simulink model "GridFormingConverter"  (R2024b)
settings: Solver=ode1be  StartTime=0.0  StopTime=simulationTime  FixedStep=gridInverter.vsm.samplingTime  MaxStep=gridInverter.vsm.samplingTime  RelTol=1e-3  AbsTol=1e-3
PreLoadFcn:
  | % Parameterize the model
  | GridFormingConverterInputParameters;
  | GFLParameters;
PostLoadFcn:
  | GridFormingConverterTestCondition;
  | GFLParameters;
undefined symbols (not defined in the file or in its folder): base, ConvCtrl, ConvPlt, DiscIntNeverNeededParam, Discrete, Fault, gcbh, GFMGFLSelect, grid, gridInverter, HMI, localSolverSampleTime, magnitude, PlantSim, scrFactorRg, scrFactorXg, sps, sps_rtmsupport, spsPLL3phModel, transformer, TransmissionLine, Trf
libraries: powerlib_extras x39, ee_lib x21, eeGeneralControl x19, nesl_utility x16, simulink x13, eeTransforms x10, fl_lib x7, spsSecondOrderFilterLib x4, spsabctodq0Lib x4, spsPower3phInstantaneousLib x3, spsMeanLib x2, eeSinGeneratorThreePhase x1
(part 2 of 6)

== system GridFormingConverter/Transformer 415 V//11 kV ==
  Circuit Breaker : ee_lib/Switches & Breakers/Circuit Breaker (Three-Phase)  R_closed=0.001 Ohm  G_open=1e-6 1/Ohm  threshold=0.5 V  breaker_behavior=ee.enum.switches.breakerBehavior.zeroCrossingEnable
      settings: InternalSimscapePortConfiguration="{\"Bottom\":[],\"Left\":[{\"id\":\"vT\",\"label\":\"vT\",\"type\":\"input\"},{\"id\":\"N1\",\"label\":\"~1\",\"type\":\"foundation.electrical.three_phase\"}],\"Right\":[{\"id\":\"N2\",\"label\":\"~2\",\"type\":\"foundation.electrical.three_phase\"}],\"Top\":[]}"
  Circuit breaker : FromWorkspace  VariableName=testCondition.circuitBreakerTripSignalProfile  SampleTime=localSolverSampleTime  Interpolate=off  OutputAfterFinalValue=Holding final value
  Filter & Sensor : Subsystem
      mask Display: image('$imagefile'); % Use "Edit Image" on toolstrip to change.
  Simulink-PS Converter : nesl_utility/Simulink-PS Converter  PhysicalDomain=network_engine_domain  SubClassName=ps_input  LeftPortType=input  RightPortType=output  PseudoPeriodic=off  Frequencies=[]  NoiseDistribution=none  NoiseParameters=[]  Unit=1  AffineConversion=off  FilteringAndDerivatives=provide  SimscapeFilterOrder=1  InputFilterTimeConstant=0.001  UdotUserProvided=0
  "Transformer " : ee_lib/Passive/Transformers/Two-Winding Transformer (Three-Phase)  SRated=base.power*1e3 A*V  FRated=gridInverter.frequency Hz  Winding1Connection=ee.enum.windingconnection.Yg  VRated1=transformer.primaryRMSVoltage V  Winding2Connection=ee.enum.windingconnection.delta1  VRated2=transformer.secondaryRMSVoltage V  CoreType=ee.enum.coretype.threelimb  pu_Rw1=transformer.PrimaryResistancePU*scrFactorRg  pu_Rw2=transformer.SecondaryResistancePU*scrFactorRg  leakage_reactance_option=ee.enum.transformer_leakage.include  pu_Xl1=transformer.PrimaryReactancePU*scrFactorXg  pu_Xl2=transformer.SecondaryReactancePU*scrFactorXg  magnetizing_resistance_option=ee.enum.transformer_magnetizingResistance.exclude  pu_Rm=500  magnetizing_reactance_option=ee.enum.transformer_magnetizingReactance.exclude  saturation_option=ee.enum.transformer_saturation.exclude  pu_Xm=500  current_data=[0, .002, 1, 2]  magnetic_flux_data=[0, 1.2, 1.5, 1.51]  pu_X0=transformer.PrimaryReactancePU*scrFactorXg*1.05  i1_specify=on  i1_priority=None  i1=[0, 0, 0] A  i1_nominal_specify=off  i1_nominal_value=1  i1_nominal_unit=A  i2_specify=on  i2_priority=None  i2=[0, 0, 0] A  i2_nominal_specify=off  i2_nominal_value=1  i2_nominal_unit=A  phi_specify=off  phi_priority=None  phi=[0, 0, 0]  phi_nominal_specify=off  phi_nominal_value=1  phi_nominal_unit=1  power_dissipated_specify=off  power_dissipated_priority=None  power_dissipated=0 W  power_dissipated_nominal_specify=off  power_dissipated_nominal_value=1  power_dissipated_nominal_unit=W
      settings: InternalSimscapePortConfiguration="{\"Bottom\":[],\"Left\":[{\"id\":\"N1\",\"label\":\"~1\",\"type\":\"foundation.electrical.three_phase\"}],\"Right\":[{\"id\":\"N2\",\"label\":\"~2\",\"type\":\"foundation.electrical.three_phase\"}],\"Top\":[]}"
  ABC1 : PMIOPort  Side=Left
  ABC2 : PMIOPort  Port=2  Side=Right
  Iabc : Outport
  Vabc : Outport  Port=2
  wires:
  Circuit breaker/1 -> Simulink-PS Converter/1  "Tripsignal"
  Filter & Sensor/1(Iabc) -> Iabc/1
  Filter & Sensor/2(Vabc) -> Vabc/1
  connections:
  "Transformer "/RConn1 -- Filter & Sensor/LConn1
  Simulink-PS Converter/RConn1 -- Circuit Breaker/LConn1
  ABC1/RConn1 -- Circuit Breaker/RConn1
  "Transformer "/LConn1 -- Circuit Breaker/LConn2
  ABC2/RConn1 -- Filter & Sensor/RConn1

== system GridFormingConverter/Transmission Line ==
  Transmission Line : ee_lib/Passive/RLC Assemblies/RLC (Three-Phase)  port_option=ee.enum.threePhasePort.composite  component_structure=ee.enum.rlc.structure.SeriesRL  R=TransmissionLine.R*scrFactorRg Ohm  L=TransmissionLine.L*scrFactorXg H  C=1e-6 F  R_parasitic=0 Ohm  G_parasitic=1e-5 1/Ohm  IL_specify=off  IL_priority=High  IL=[0, 0, 0] A  IL_nominal_specify=off  IL_nominal_value=1  IL_nominal_unit=A  VC_specify=off  VC_priority=High  VC=[0, 0, 0] V  VC_nominal_specify=off  VC_nominal_value=1  VC_nominal_unit=V
      settings: InternalSimscapePortConfiguration="{\"Bottom\":[],\"Left\":[{\"id\":\"N1\",\"label\":\"~1\",\"type\":\"foundation.electrical.three_phase\"}],\"Right\":[{\"id\":\"N2\",\"label\":\"~2\",\"type\":\"foundation.electrical.three_phase\"}],\"Top\":[]}"
  ABC1 : PMIOPort  Side=Left
  ABC2 : PMIOPort  Port=2  Side=Right
  connections:
  Transmission Line/RConn1 -- ABC2/RConn1
  ABC1/RConn1 -- Transmission Line/LConn1

== system GridFormingConverter/BusCalculations/Complex2Phasor ==
  complex : Inport
  Bus Creator1 : BusCreator  Inputs=3
  Bus Creator2 : BusCreator  Inputs=2
  Bus Creator3 : BusCreator  Inputs=2
  Bus Creator5 : BusCreator  Inputs=2
  Complex to Magnitude-Angle3 : ComplexToMagnitudeAngle
  Demux2 : Demux  Outputs=3
  Demux3 : Demux  Outputs=3
  Gain : Gain  Gain=180/pi
  Phasor : Outport
  wires:
  complex/1 -> Complex to Magnitude-Angle3/1
  Demux2/3 -> Bus Creator3/1  "mag"
  Complex to Magnitude-Angle3/1 -> Demux2/1
  Demux3/2 -> Bus Creator5/2  "phase"
  Demux2/1 -> Bus Creator2/1  "mag"
  Complex to Magnitude-Angle3/2 -> Gain/1
  Demux2/2 -> Bus Creator5/1  "mag"
  Demux3/1 -> Bus Creator2/2  "phase"
  Demux3/3 -> Bus Creator3/2  "phase"
  Bus Creator2/1 -> Bus Creator1/1  "a"
  Bus Creator5/1 -> Bus Creator1/2  "b"
  Bus Creator3/1 -> Bus Creator1/3  "c"
  Bus Creator1/1 -> Phasor/1  "Phasor"
  Gain/1 -> Demux3/1

== system GridFormingConverter/BusCalculations/Complex2Phasor1 ==
  complex : Inport
  Bus Creator1 : BusCreator  Inputs=3
  Bus Creator2 : BusCreator  Inputs=2
  Bus Creator3 : BusCreator  Inputs=2
  Bus Creator5 : BusCreator  Inputs=2
  Complex to Magnitude-Angle3 : ComplexToMagnitudeAngle
  Demux2 : Demux  Outputs=3
  Demux3 : Demux  Outputs=3
  Gain : Gain  Gain=180/pi
  Phasor : Outport
  wires:
  Bus Creator1/1 -> Phasor/1  "Phasor"
  Bus Creator3/1 -> Bus Creator1/3  "c"
  Bus Creator5/1 -> Bus Creator1/2  "b"
  Bus Creator2/1 -> Bus Creator1/1  "a"
  Demux3/3 -> Bus Creator3/2  "phase"
  Demux3/1 -> Bus Creator2/2  "phase"
  Demux2/2 -> Bus Creator5/1  "mag"
  Complex to Magnitude-Angle3/2 -> Gain/1
  Demux2/1 -> Bus Creator2/1  "mag"
  Demux3/2 -> Bus Creator5/2  "phase"
  Complex to Magnitude-Angle3/1 -> Demux2/1
  Demux2/3 -> Bus Creator3/1  "mag"
  complex/1 -> Complex to Magnitude-Angle3/1
  Gain/1 -> Demux3/1

== system GridFormingConverter/BusCalculations/Measurement Unit (Phasor Computation) ==
  Vabc(t) : Inport  PortDimensions=3
  Iabc(t) : Inport  Port=2  PortDimensions=3
  Demux : Demux  Outputs=3
      settings: DisplayOption=none
  Demux1 : Demux  Outputs=3
      settings: DisplayOption=none
  Discrete Fourier(A) : Subsystem  AncestorBlock=|  mask(Discrete Fourier){Freq=Freq, n=1, Par_Init=[0 0], Ts=Ts}
      | powerlib_extras/Discrete
      | Measurements/Discrete 
      | Fourier
      mask prompts: Freq "Fundamental frequency (Hz):"; n "Harmonic n (0=DC; 1=fundamental; 2=2nd harm;  ...):"; Par_Init "Initial input: [ Mag  Phase(degrees) ]"; Ts "Sample time:"
      mask help:
      | This block computes the fundamental value of the input signal over a running window of one cycle of the specified fundamental frequency. First and second outputs return respectively the magnitude and phase (degrees) of the fundamental.
      | For the first cycle of simulation, the ouputs are held constant to the value specified by the parameter "Initial input".
      mask init:
      | k=2-(n==0);
      | SamplesPerCycle=1/Freq/Ts;
      | RoundSamplesPerCycle=round(SamplesPerCycle);
      | Delay=RoundSamplesPerCycle*Ts - Ts/2;
      | Correction=SamplesPerCycle/RoundSamplesPerCycle - 1;
      | Real_Init=Par_Init(1)*cos(pi/180*Par_Init(2));
      | Imag_Init=Par_Init(1)*sin(pi/180*Par_Init(2));
  "Discrete Fourier(A) " : Subsystem  AncestorBlock=|  mask(Discrete Fourier){Freq=Freq, n=1, Par_Init=[0 0], Ts=Ts}
      | powerlib_extras/Discrete
      | Measurements/Discrete 
      | Fourier
      mask prompts: Freq "Fundamental frequency (Hz):"; n "Harmonic n (0=DC; 1=fundamental; 2=2nd harm;  ...):"; Par_Init "Initial input: [ Mag  Phase(degrees) ]"; Ts "Sample time:"
      mask help:
      | This block computes the fundamental value of the input signal over a running window of one cycle of the specified fundamental frequency. First and second outputs return respectively the magnitude and phase (degrees) of the fundamental.
      | For the first cycle of simulation, the ouputs are held constant to the value specified by the parameter "Initial input".
      mask init: same as GridFormingConverter/BusCalculations/Measurement Unit (Phasor Computation)/Discrete Fourier(A)
  Discrete Fourier(B) : Subsystem  AncestorBlock=|  mask(Discrete Fourier){Freq=Freq, n=1, Par_Init=[0 -120], Ts=Ts}
      | powerlib_extras/Discrete
      | Measurements/Discrete 
      | Fourier
      mask prompts: Freq "Fundamental frequency (Hz):"; n "Harmonic n (0=DC; 1=fundamental; 2=2nd harm;  ...):"; Par_Init "Initial input: [ Mag  Phase(degrees) ]"; Ts "Sample time:"
      mask help:
      | This block computes the fundamental value of the input signal over a running window of one cycle of the specified fundamental frequency. First and second outputs return respectively the magnitude and phase (degrees) of the fundamental.
      | For the first cycle of simulation, the ouputs are held constant to the value specified by the parameter "Initial input".
      mask init: same as GridFormingConverter/BusCalculations/Measurement Unit (Phasor Computation)/Discrete Fourier(A)
  "Discrete Fourier(B) " : Subsystem  AncestorBlock=|  mask(Discrete Fourier){Freq=Freq, n=1, Par_Init=[0 -120], Ts=Ts}
      | powerlib_extras/Discrete
      | Measurements/Discrete 
      | Fourier
      mask prompts: Freq "Fundamental frequency (Hz):"; n "Harmonic n (0=DC; 1=fundamental; 2=2nd harm;  ...):"; Par_Init "Initial input: [ Mag  Phase(degrees) ]"; Ts "Sample time:"
      mask help:
      | This block computes the fundamental value of the input signal over a running window of one cycle of the specified fundamental frequency. First and second outputs return respectively the magnitude and phase (degrees) of the fundamental.
      | For the first cycle of simulation, the ouputs are held constant to the value specified by the parameter "Initial input".
      mask init: same as GridFormingConverter/BusCalculations/Measurement Unit (Phasor Computation)/Discrete Fourier(A)
  Discrete Fourier(C) : Subsystem  AncestorBlock=|  mask(Discrete Fourier){Freq=Freq, n=1, Par_Init=[0 120], Ts=Ts}
      | powerlib_extras/Discrete
      | Measurements/Discrete 
      | Fourier
      mask prompts: Freq "Fundamental frequency (Hz):"; n "Harmonic n (0=DC; 1=fundamental; 2=2nd harm;  ...):"; Par_Init "Initial input: [ Mag  Phase(degrees) ]"; Ts "Sample time:"
      mask help:
      | This block computes the fundamental value of the input signal over a running window of one cycle of the specified fundamental frequency. First and second outputs return respectively the magnitude and phase (degrees) of the fundamental.
      | For the first cycle of simulation, the ouputs are held constant to the value specified by the parameter "Initial input".
      mask init: same as GridFormingConverter/BusCalculations/Measurement Unit (Phasor Computation)/Discrete Fourier(A)
  "Discrete Fourier(C) " : Subsystem  AncestorBlock=|  mask(Discrete Fourier){Freq=Freq, n=1, Par_Init=[0 120], Ts=Ts}
      | powerlib_extras/Discrete
      | Measurements/Discrete 
      | Fourier
      mask prompts: Freq "Fundamental frequency (Hz):"; n "Harmonic n (0=DC; 1=fundamental; 2=2nd harm;  ...):"; Par_Init "Initial input: [ Mag  Phase(degrees) ]"; Ts "Sample time:"
      mask help:
      | This block computes the fundamental value of the input signal over a running window of one cycle of the specified fundamental frequency. First and second outputs return respectively the magnitude and phase (degrees) of the fundamental.
      | For the first cycle of simulation, the ouputs are held constant to the value specified by the parameter "Initial input".
      mask init: same as GridFormingConverter/BusCalculations/Measurement Unit (Phasor Computation)/Discrete Fourier(A)
  Mux : Mux  Inputs=3
  Mux1 : Mux  Inputs=3
  Vabc_Fund : Outport
  " Iabc_Fund" : Outport  Port=2
  wires:
  "Discrete Fourier(C) "/1(Fund) -> Mux1/3
  "Discrete Fourier(B) "/1(Fund) -> Mux1/2
  "Discrete Fourier(A) "/1(Fund) -> Mux1/1
  Mux1/1 -> " Iabc_Fund"/1
  Iabc(t)/1 -> Demux1/1
  Demux1/3 -> "Discrete Fourier(C) "/1(In)
  Demux1/2 -> "Discrete Fourier(B) "/1(In)
  Demux1/1 -> "Discrete Fourier(A) "/1(In)
  Mux/1 -> Vabc_Fund/1
  Discrete Fourier(C)/1(Fund) -> Mux/3
  Discrete Fourier(B)/1(Fund) -> Mux/2
  Discrete Fourier(A)/1(Fund) -> Mux/1
  Demux/3 -> Discrete Fourier(C)/1(In)
  Demux/2 -> Discrete Fourier(B)/1(In)
  Vabc(t)/1 -> Demux/1
  Demux/1 -> Discrete Fourier(A)/1(In)

== system GridFormingConverter/BusCalculations/SymmetricalComponentsCalc ==
  abc : Inport
  Bus Creator{,1..4,7..8} (7 alike) : BusCreator  Inputs=3
  Bus Creator5 : BusCreator  Inputs=2
  Bus Creator6 : BusCreator  Inputs=2
  Bus Creator9 : BusCreator  Inputs=2
  Complex to Magnitude-Angle1 : ComplexToMagnitudeAngle
  Complex to Magnitude-Angle2 : ComplexToMagnitudeAngle
  Complex to Magnitude-Angle3 : ComplexToMagnitudeAngle
  Demux{,1..5} (6 alike) : Demux  Outputs=3
  Gain : Gain  Gain=[exp(1i*4*pi/3) 0 0; 0 exp(1i*2*pi/3) 0; 0 0 1]  Multiplication=Matrix(K*u)
  Gain1 : Gain  Gain=[exp(1i*2*pi/3) 0 0; 0 exp(1i*4*pi/3) 0; 0 0 1]  Multiplication=Matrix(K*u)
  Gain2 : Gain  Gain=180/pi
  Gain3 : Gain  Gain=180/pi
  Gain4 : Gain  Gain=180/pi
  Symmetrical-Components Transform1 : eeTransforms/Symmetrical-Components Transform  PowerInvariant=off
  ABC+-0 : Outport
  wires:
  Demux/2 -> Bus Creator3/2  "neg"
  Complex to Magnitude-Angle3/2 -> Gain2/1
  Demux/1 -> Bus Creator3/1  "pos"
  Symmetrical-Components Transform1/1 -> Complex to Magnitude-Angle3/1, Gain/1, Gain1/1
  Demux/3 -> Bus Creator3/3  "zero"
  Bus Creator3/1 -> Bus Creator5/1  "mag"
  Complex to Magnitude-Angle3/1 -> Demux/1
  Bus Creator4/1 -> Bus Creator5/2  "phase"
  abc/1 -> Symmetrical-Components Transform1/1
  Bus Creator5/1 -> Bus Creator/1  "A"
  Bus Creator6/1 -> Bus Creator/2  "B"
  Bus Creator2/1 -> Bus Creator6/2  "phase"
  Complex to Magnitude-Angle1/1 -> Demux2/1
  Bus Creator1/1 -> Bus Creator6/1  "mag"
  Complex to Magnitude-Angle1/2 -> Gain3/1
  Gain/1 -> Complex to Magnitude-Angle1/1
  Complex to Magnitude-Angle2/2 -> Gain4/1
  Bus Creator7/1 -> Bus Creator9/1  "mag"
  Complex to Magnitude-Angle2/1 -> Demux4/1
  Bus Creator8/1 -> Bus Creator9/2  "phase"
  Bus Creator9/1 -> Bus Creator/3  "C"
  Gain1/1 -> Complex to Magnitude-Angle2/1
  Bus Creator/1 -> ABC+-0/1
  Demux1/1 -> Bus Creator4/1  "pos"
  Demux1/3 -> Bus Creator4/3  "zero"
  Demux1/2 -> Bus Creator4/2  "neg"
  Demux2/2 -> Bus Creator1/2  "neg"
  Demux2/3 -> Bus Creator1/3  "zero"
  Demux2/1 -> Bus Creator1/1  "pos"
  Demux3/2 -> Bus Creator2/2  "neg"
  Demux3/3 -> Bus Creator2/3  "zero"
  Demux3/1 -> Bus Creator2/1  "pos"
  Demux4/2 -> Bus Creator7/2  "neg"
  Demux4/3 -> Bus Creator7/3  "zero"
  Demux4/1 -> Bus Creator7/1  "pos"
  Demux5/2 -> Bus Creator8/2  "neg"
  Demux5/3 -> Bus Creator8/3  "zero"
  Demux5/1 -> Bus Creator8/1  "pos"
  Gain2/1 -> Demux1/1
  Gain3/1 -> Demux3/1
  Gain4/1 -> Demux5/1

== system GridFormingConverter/BusCalculations/SymmetricalComponentsCalc1 ==
  abc : Inport
  Bus Creator{,1..4,7..8} (7 alike) : BusCreator  Inputs=3
  Bus Creator5 : BusCreator  Inputs=2
  Bus Creator6 : BusCreator  Inputs=2
  Bus Creator9 : BusCreator  Inputs=2
  Complex to Magnitude-Angle1 : ComplexToMagnitudeAngle
  Complex to Magnitude-Angle2 : ComplexToMagnitudeAngle
  Complex to Magnitude-Angle3 : ComplexToMagnitudeAngle
  Demux{,1..5} (6 alike) : Demux  Outputs=3
  Gain : Gain  Gain=[exp(1i*4*pi/3) 0 0; 0 exp(1i*2*pi/3) 0; 0 0 1]  Multiplication=Matrix(K*u)
  Gain1 : Gain  Gain=[exp(1i*2*pi/3) 0 0; 0 exp(1i*4*pi/3) 0; 0 0 1]  Multiplication=Matrix(K*u)
  Gain2 : Gain  Gain=180/pi
  Gain3 : Gain  Gain=180/pi
  Gain4 : Gain  Gain=180/pi
  Symmetrical-Components Transform1 : eeTransforms/Symmetrical-Components Transform  PowerInvariant=off
  ABC+-0 : Outport
  wires:
  Gain4/1 -> Demux5/1
  Gain3/1 -> Demux3/1
  Gain2/1 -> Demux1/1
  Demux5/1 -> Bus Creator8/1  "pos"
  Demux5/3 -> Bus Creator8/3  "zero"
  Demux5/2 -> Bus Creator8/2  "neg"
  Demux4/1 -> Bus Creator7/1  "pos"
  Demux4/3 -> Bus Creator7/3  "zero"
  Demux4/2 -> Bus Creator7/2  "neg"
  Demux3/1 -> Bus Creator2/1  "pos"
  Demux3/3 -> Bus Creator2/3  "zero"
  Demux3/2 -> Bus Creator2/2  "neg"
  Demux2/1 -> Bus Creator1/1  "pos"
  Demux2/3 -> Bus Creator1/3  "zero"
  Demux2/2 -> Bus Creator1/2  "neg"
  Demux1/2 -> Bus Creator4/2  "neg"
  Demux1/3 -> Bus Creator4/3  "zero"
  Demux1/1 -> Bus Creator4/1  "pos"
  Bus Creator/1 -> ABC+-0/1
  Gain1/1 -> Complex to Magnitude-Angle2/1
  Bus Creator9/1 -> Bus Creator/3  "C"
  Bus Creator8/1 -> Bus Creator9/2  "phase"
  Complex to Magnitude-Angle2/1 -> Demux4/1
  Bus Creator7/1 -> Bus Creator9/1  "mag"
  Complex to Magnitude-Angle2/2 -> Gain4/1
  Gain/1 -> Complex to Magnitude-Angle1/1
  Complex to Magnitude-Angle1/2 -> Gain3/1
  Bus Creator1/1 -> Bus Creator6/1  "mag"
  Complex to Magnitude-Angle1/1 -> Demux2/1
  Bus Creator2/1 -> Bus Creator6/2  "phase"
  Bus Creator6/1 -> Bus Creator/2  "B"
  Bus Creator5/1 -> Bus Creator/1  "A"
  abc/1 -> Symmetrical-Components Transform1/1
  Bus Creator4/1 -> Bus Creator5/2  "phase"
  Complex to Magnitude-Angle3/1 -> Demux/1
  Bus Creator3/1 -> Bus Creator5/1  "mag"
  Demux/3 -> Bus Creator3/3  "zero"
  Symmetrical-Components Transform1/1 -> Gain1/1, Gain/1, Complex to Magnitude-Angle3/1
  Demux/1 -> Bus Creator3/1  "pos"
  Complex to Magnitude-Angle3/2 -> Gain2/1
  Demux/2 -> Bus Creator3/2  "neg"

== system GridFormingConverter/BusCalculations1/Complex2Phasor ==
  complex : Inport
  Bus Creator1 : BusCreator  Inputs=3
  Bus Creator2 : BusCreator  Inputs=2
  Bus Creator3 : BusCreator  Inputs=2
  Bus Creator5 : BusCreator  Inputs=2
  Complex to Magnitude-Angle3 : ComplexToMagnitudeAngle
  Demux2 : Demux  Outputs=3
  Demux3 : Demux  Outputs=3
  Gain : Gain  Gain=180/pi
  Phasor : Outport
  wires:
  Gain/1 -> Demux3/1
  Bus Creator1/1 -> Phasor/1  "Phasor"
  Bus Creator3/1 -> Bus Creator1/3  "c"
  Bus Creator5/1 -> Bus Creator1/2  "b"
  Bus Creator2/1 -> Bus Creator1/1  "a"
  Demux3/3 -> Bus Creator3/2  "phase"
  Demux3/1 -> Bus Creator2/2  "phase"
  Demux2/2 -> Bus Creator5/1  "mag"
  Complex to Magnitude-Angle3/2 -> Gain/1
  Demux2/1 -> Bus Creator2/1  "mag"
  Demux3/2 -> Bus Creator5/2  "phase"
  Complex to Magnitude-Angle3/1 -> Demux2/1
  Demux2/3 -> Bus Creator3/1  "mag"
  complex/1 -> Complex to Magnitude-Angle3/1

== system GridFormingConverter/BusCalculations1/Complex2Phasor1 ==
  complex : Inport
  Bus Creator1 : BusCreator  Inputs=3
  Bus Creator2 : BusCreator  Inputs=2
  Bus Creator3 : BusCreator  Inputs=2
  Bus Creator5 : BusCreator  Inputs=2
  Complex to Magnitude-Angle3 : ComplexToMagnitudeAngle
  Demux2 : Demux  Outputs=3
  Demux3 : Demux  Outputs=3
  Gain : Gain  Gain=180/pi
  Phasor : Outport
  wires:
  Gain/1 -> Demux3/1
  complex/1 -> Complex to Magnitude-Angle3/1
  Demux2/3 -> Bus Creator3/1  "mag"
  Complex to Magnitude-Angle3/1 -> Demux2/1
  Demux3/2 -> Bus Creator5/2  "phase"
  Demux2/1 -> Bus Creator2/1  "mag"
  Complex to Magnitude-Angle3/2 -> Gain/1
  Demux2/2 -> Bus Creator5/1  "mag"
  Demux3/1 -> Bus Creator2/2  "phase"
  Demux3/3 -> Bus Creator3/2  "phase"
  Bus Creator2/1 -> Bus Creator1/1  "a"
  Bus Creator5/1 -> Bus Creator1/2  "b"
  Bus Creator3/1 -> Bus Creator1/3  "c"
  Bus Creator1/1 -> Phasor/1  "Phasor"

== system GridFormingConverter/BusCalculations1/Measurement Unit (Phasor Computation) ==
  Vabc(t) : Inport  PortDimensions=3
  Iabc(t) : Inport  Port=2  PortDimensions=3
  Demux : Demux  Outputs=3
      settings: DisplayOption=none
  Demux1 : Demux  Outputs=3
      settings: DisplayOption=none
  Discrete Fourier(A) : Subsystem  AncestorBlock=|  mask(Discrete Fourier){Freq=Freq, n=1, Par_Init=[0 0], Ts=Ts}
      | powerlib_extras/Discrete
      | Measurements/Discrete 
      | Fourier
      mask prompts: Freq "Fundamental frequency (Hz):"; n "Harmonic n (0=DC; 1=fundamental; 2=2nd harm;  ...):"; Par_Init "Initial input: [ Mag  Phase(degrees) ]"; Ts "Sample time:"
      mask help:
      | This block computes the fundamental value of the input signal over a running window of one cycle of the specified fundamental frequency. First and second outputs return respectively the magnitude and phase (degrees) of the fundamental.
      | For the first cycle of simulation, the ouputs are held constant to the value specified by the parameter "Initial input".
      mask init: same as GridFormingConverter/BusCalculations/Measurement Unit (Phasor Computation)/Discrete Fourier(A)
  "Discrete Fourier(A) " : Subsystem  AncestorBlock=|  mask(Discrete Fourier){Freq=Freq, n=1, Par_Init=[0 0], Ts=Ts}
      | powerlib_extras/Discrete
      | Measurements/Discrete 
      | Fourier
      mask prompts: Freq "Fundamental frequency (Hz):"; n "Harmonic n (0=DC; 1=fundamental; 2=2nd harm;  ...):"; Par_Init "Initial input: [ Mag  Phase(degrees) ]"; Ts "Sample time:"
      mask help:
      | This block computes the fundamental value of the input signal over a running window of one cycle of the specified fundamental frequency. First and second outputs return respectively the magnitude and phase (degrees) of the fundamental.
      | For the first cycle of simulation, the ouputs are held constant to the value specified by the parameter "Initial input".
      mask init: same as GridFormingConverter/BusCalculations/Measurement Unit (Phasor Computation)/Discrete Fourier(A)
  Discrete Fourier(B) : Subsystem  AncestorBlock=|  mask(Discrete Fourier){Freq=Freq, n=1, Par_Init=[0 -120], Ts=Ts}
      | powerlib_extras/Discrete
      | Measurements/Discrete 
      | Fourier
      mask prompts: Freq "Fundamental frequency (Hz):"; n "Harmonic n (0=DC; 1=fundamental; 2=2nd harm;  ...):"; Par_Init "Initial input: [ Mag  Phase(degrees) ]"; Ts "Sample time:"
      mask help:
      | This block computes the fundamental value of the input signal over a running window of one cycle of the specified fundamental frequency. First and second outputs return respectively the magnitude and phase (degrees) of the fundamental.
      | For the first cycle of simulation, the ouputs are held constant to the value specified by the parameter "Initial input".
      mask init: same as GridFormingConverter/BusCalculations/Measurement Unit (Phasor Computation)/Discrete Fourier(A)
  "Discrete Fourier(B) " : Subsystem  AncestorBlock=|  mask(Discrete Fourier){Freq=Freq, n=1, Par_Init=[0 -120], Ts=Ts}
      | powerlib_extras/Discrete
      | Measurements/Discrete 
      | Fourier
      mask prompts: Freq "Fundamental frequency (Hz):"; n "Harmonic n (0=DC; 1=fundamental; 2=2nd harm;  ...):"; Par_Init "Initial input: [ Mag  Phase(degrees) ]"; Ts "Sample time:"
      mask help:
      | This block computes the fundamental value of the input signal over a running window of one cycle of the specified fundamental frequency. First and second outputs return respectively the magnitude and phase (degrees) of the fundamental.
      | For the first cycle of simulation, the ouputs are held constant to the value specified by the parameter "Initial input".
      mask init: same as GridFormingConverter/BusCalculations/Measurement Unit (Phasor Computation)/Discrete Fourier(A)
  Discrete Fourier(C) : Subsystem  AncestorBlock=|  mask(Discrete Fourier){Freq=Freq, n=1, Par_Init=[0 120], Ts=Ts}
      | powerlib_extras/Discrete
      | Measurements/Discrete 
      | Fourier
      mask prompts: Freq "Fundamental frequency (Hz):"; n "Harmonic n (0=DC; 1=fundamental; 2=2nd harm;  ...):"; Par_Init "Initial input: [ Mag  Phase(degrees) ]"; Ts "Sample time:"
      mask help:
      | This block computes the fundamental value of the input signal over a running window of one cycle of the specified fundamental frequency. First and second outputs return respectively the magnitude and phase (degrees) of the fundamental.
      | For the first cycle of simulation, the ouputs are held constant to the value specified by the parameter "Initial input".
      mask init: same as GridFormingConverter/BusCalculations/Measurement Unit (Phasor Computation)/Discrete Fourier(A)
  "Discrete Fourier(C) " : Subsystem  AncestorBlock=|  mask(Discrete Fourier){Freq=Freq, n=1, Par_Init=[0 120], Ts=Ts}
      | powerlib_extras/Discrete
      | Measurements/Discrete 
      | Fourier
      mask prompts: Freq "Fundamental frequency (Hz):"; n "Harmonic n (0=DC; 1=fundamental; 2=2nd harm;  ...):"; Par_Init "Initial input: [ Mag  Phase(degrees) ]"; Ts "Sample time:"
      mask help:
      | This block computes the fundamental value of the input signal over a running window of one cycle of the specified fundamental frequency. First and second outputs return respectively the magnitude and phase (degrees) of the fundamental.
      | For the first cycle of simulation, the ouputs are held constant to the value specified by the parameter "Initial input".
      mask init: same as GridFormingConverter/BusCalculations/Measurement Unit (Phasor Computation)/Discrete Fourier(A)
  Mux : Mux  Inputs=3
  Mux1 : Mux  Inputs=3
  Vabc_Fund : Outport
  " Iabc_Fund" : Outport  Port=2
  wires:
  Demux/1 -> Discrete Fourier(A)/1(In)
  Vabc(t)/1 -> Demux/1
  Demux/2 -> Discrete Fourier(B)/1(In)
  Demux/3 -> Discrete Fourier(C)/1(In)
  Discrete Fourier(A)/1(Fund) -> Mux/1
  Discrete Fourier(B)/1(Fund) -> Mux/2
  Discrete Fourier(C)/1(Fund) -> Mux/3
  Mux/1 -> Vabc_Fund/1
  Demux1/1 -> "Discrete Fourier(A) "/1(In)
  Demux1/2 -> "Discrete Fourier(B) "/1(In)
  Demux1/3 -> "Discrete Fourier(C) "/1(In)
  Iabc(t)/1 -> Demux1/1
  Mux1/1 -> " Iabc_Fund"/1
  "Discrete Fourier(A) "/1(Fund) -> Mux1/1
  "Discrete Fourier(B) "/1(Fund) -> Mux1/2
  "Discrete Fourier(C) "/1(Fund) -> Mux1/3

== system GridFormingConverter/BusCalculations1/SymmetricalComponentsCalc ==
  abc : Inport
  Bus Creator{,1..4,7..8} (7 alike) : BusCreator  Inputs=3
  Bus Creator5 : BusCreator  Inputs=2
  Bus Creator6 : BusCreator  Inputs=2
  Bus Creator9 : BusCreator  Inputs=2
  Complex to Magnitude-Angle1 : ComplexToMagnitudeAngle
  Complex to Magnitude-Angle2 : ComplexToMagnitudeAngle
  Complex to Magnitude-Angle3 : ComplexToMagnitudeAngle
  Demux{,1..5} (6 alike) : Demux  Outputs=3
  Gain : Gain  Gain=[exp(1i*4*pi/3) 0 0; 0 exp(1i*2*pi/3) 0; 0 0 1]  Multiplication=Matrix(K*u)
  Gain1 : Gain  Gain=[exp(1i*2*pi/3) 0 0; 0 exp(1i*4*pi/3) 0; 0 0 1]  Multiplication=Matrix(K*u)
  Gain2 : Gain  Gain=180/pi
  Gain3 : Gain  Gain=180/pi
  Gain4 : Gain  Gain=180/pi
  Symmetrical-Components Transform1 : eeTransforms/Symmetrical-Components Transform  PowerInvariant=off
  ABC+-0 : Outport
  wires:
  Gain4/1 -> Demux5/1
  Gain3/1 -> Demux3/1
  Gain2/1 -> Demux1/1
  Demux5/1 -> Bus Creator8/1  "pos"
  Demux5/3 -> Bus Creator8/3  "zero"
  Demux5/2 -> Bus Creator8/2  "neg"
  Demux4/1 -> Bus Creator7/1  "pos"
  Demux4/3 -> Bus Creator7/3  "zero"
  Demux4/2 -> Bus Creator7/2  "neg"
  Demux3/1 -> Bus Creator2/1  "pos"
  Demux3/3 -> Bus Creator2/3  "zero"
  Demux3/2 -> Bus Creator2/2  "neg"
  Demux2/1 -> Bus Creator1/1  "pos"
  Demux2/3 -> Bus Creator1/3  "zero"
  Demux2/2 -> Bus Creator1/2  "neg"
  Demux1/2 -> Bus Creator4/2  "neg"
  Demux1/3 -> Bus Creator4/3  "zero"
  Demux1/1 -> Bus Creator4/1  "pos"
  Bus Creator/1 -> ABC+-0/1
  Gain1/1 -> Complex to Magnitude-Angle2/1
  Bus Creator9/1 -> Bus Creator/3  "C"
  Bus Creator8/1 -> Bus Creator9/2  "phase"
  Complex to Magnitude-Angle2/1 -> Demux4/1
  Bus Creator7/1 -> Bus Creator9/1  "mag"
  Complex to Magnitude-Angle2/2 -> Gain4/1
  Gain/1 -> Complex to Magnitude-Angle1/1
  Complex to Magnitude-Angle1/2 -> Gain3/1
  Bus Creator1/1 -> Bus Creator6/1  "mag"
  Complex to Magnitude-Angle1/1 -> Demux2/1
  Bus Creator2/1 -> Bus Creator6/2  "phase"
  Bus Creator6/1 -> Bus Creator/2  "B"
  Bus Creator5/1 -> Bus Creator/1  "A"
  abc/1 -> Symmetrical-Components Transform1/1
  Bus Creator4/1 -> Bus Creator5/2  "phase"
  Complex to Magnitude-Angle3/1 -> Demux/1
  Bus Creator3/1 -> Bus Creator5/1  "mag"
  Demux/3 -> Bus Creator3/3  "zero"
  Symmetrical-Components Transform1/1 -> Gain1/1, Gain/1, Complex to Magnitude-Angle3/1
  Demux/1 -> Bus Creator3/1  "pos"
  Complex to Magnitude-Angle3/2 -> Gain2/1
  Demux/2 -> Bus Creator3/2  "neg"

== system GridFormingConverter/BusCalculations1/SymmetricalComponentsCalc1 ==
  abc : Inport
  Bus Creator{,1..4,7..8} (7 alike) : BusCreator  Inputs=3
  Bus Creator5 : BusCreator  Inputs=2
  Bus Creator6 : BusCreator  Inputs=2
  Bus Creator9 : BusCreator  Inputs=2
  Complex to Magnitude-Angle1 : ComplexToMagnitudeAngle
  Complex to Magnitude-Angle2 : ComplexToMagnitudeAngle
  Complex to Magnitude-Angle3 : ComplexToMagnitudeAngle
  Demux{,1..5} (6 alike) : Demux  Outputs=3
  Gain : Gain  Gain=[exp(1i*4*pi/3) 0 0; 0 exp(1i*2*pi/3) 0; 0 0 1]  Multiplication=Matrix(K*u)
  Gain1 : Gain  Gain=[exp(1i*2*pi/3) 0 0; 0 exp(1i*4*pi/3) 0; 0 0 1]  Multiplication=Matrix(K*u)
  Gain2 : Gain  Gain=180/pi
  Gain3 : Gain  Gain=180/pi
  Gain4 : Gain  Gain=180/pi
  Symmetrical-Components Transform1 : eeTransforms/Symmetrical-Components Transform  PowerInvariant=off
  ABC+-0 : Outport
  wires:
  Demux/2 -> Bus Creator3/2  "neg"
  Complex to Magnitude-Angle3/2 -> Gain2/1
  Demux/1 -> Bus Creator3/1  "pos"
  Symmetrical-Components Transform1/1 -> Complex to Magnitude-Angle3/1, Gain/1, Gain1/1
  Demux/3 -> Bus Creator3/3  "zero"
  Bus Creator3/1 -> Bus Creator5/1  "mag"
  Complex to Magnitude-Angle3/1 -> Demux/1
  Bus Creator4/1 -> Bus Creator5/2  "phase"
  abc/1 -> Symmetrical-Components Transform1/1
  Bus Creator5/1 -> Bus Creator/1  "A"
  Bus Creator6/1 -> Bus Creator/2  "B"
  Bus Creator2/1 -> Bus Creator6/2  "phase"
  Complex to Magnitude-Angle1/1 -> Demux2/1
  Bus Creator1/1 -> Bus Creator6/1  "mag"
  Complex to Magnitude-Angle1/2 -> Gain3/1
  Gain/1 -> Complex to Magnitude-Angle1/1
  Complex to Magnitude-Angle2/2 -> Gain4/1
  Bus Creator7/1 -> Bus Creator9/1  "mag"
  Complex to Magnitude-Angle2/1 -> Demux4/1
  Bus Creator8/1 -> Bus Creator9/2  "phase"
  Bus Creator9/1 -> Bus Creator/3  "C"
  Gain1/1 -> Complex to Magnitude-Angle2/1
  Bus Creator/1 -> ABC+-0/1
  Demux1/1 -> Bus Creator4/1  "pos"
  Demux1/3 -> Bus Creator4/3  "zero"
  Demux1/2 -> Bus Creator4/2  "neg"
  Demux2/2 -> Bus Creator1/2  "neg"
  Demux2/3 -> Bus Creator1/3  "zero"
  Demux2/1 -> Bus Creator1/1  "pos"
  Demux3/2 -> Bus Creator2/2  "neg"
  Demux3/3 -> Bus Creator2/3  "zero"
  Demux3/1 -> Bus Creator2/1  "pos"
  Demux4/2 -> Bus Creator7/2  "neg"
  Demux4/3 -> Bus Creator7/3  "zero"
  Demux4/1 -> Bus Creator7/1  "pos"
  Demux5/2 -> Bus Creator8/2  "neg"
  Demux5/3 -> Bus Creator8/3  "zero"
  Demux5/1 -> Bus Creator8/1  "pos"
  Gain2/1 -> Demux1/1
  Gain3/1 -> Demux3/1
  Gain4/1 -> Demux5/1

== system GridFormingConverter/Grid/Filter & Sensor ==
  Current Sensor (Three-Phase) : ee_lib/Sensors & Transducers/Current Sensor (Three-Phase)
  Electrical Reference1 : fl_lib/Electrical/Electrical Elements/Electrical Reference
  Low-Pass Filter (Discrete or Continuous)1 : eeGeneralControl/Low-Pass Filter (Discrete or Continuous)  K=1  T=1/(200*gridInverter.frequency)  B=inf  A=-inf  init_option=Specify as parameter  x0=0  Ts=gridInverter.controller.VoltageControlSampleTime
  Low-Pass Filter (Discrete or Continuous)2 : eeGeneralControl/Low-Pass Filter (Discrete or Continuous)  K=1  T=1/(200*gridInverter.frequency)  B=inf  A=-inf  init_option=Specify as parameter  x0=0  Ts=gridInverter.controller.VoltageControlSampleTime
  Neutral Port (Three-Phase) : ee_lib/Connectors & References/Neutral Port (Three-Phase)  G_parasitic=1e-12 1/Ohm
      settings: InternalSimscapePortConfiguration="{\"Bottom\":[],\"Left\":[{\"id\":\"N\",\"label\":\"~\",\"type\":\"foundation.electrical.three_phase\"}],\"Right\":[{\"id\":\"n\",\"label\":\"n\",\"type\":\"foundation.electrical.electrical\"}],\"Top\":[]}"
  PS-Simulink Converter : nesl_utility/PS-Simulink Converter  PhysicalDomain=network_engine_domain  SubClassName=ps_output  LeftPortType=input  RightPortType=output  PseudoPeriodic=off  Frequencies=[]  VectorFormat=inherit  Unit=inherit  AffineConversion=off
  PS-Simulink Converter1 : nesl_utility/PS-Simulink Converter  PhysicalDomain=network_engine_domain  SubClassName=ps_output  LeftPortType=input  RightPortType=output  PseudoPeriodic=off  Frequencies=[]  VectorFormat=inherit  Unit=inherit  AffineConversion=off
  Phase Voltage Sensor (Three-Phase) : ee_lib/Sensors & Transducers/Phase Voltage Sensor (Three-Phase)
  Inabc : PMIOPort  Side=Left
  Opabc : PMIOPort  Port=2  Side=Right
  Iabc : Outport
  Vabc : Outport  Port=2
  wires:
  PS-Simulink Converter1/1 -> Low-Pass Filter (Discrete or Continuous)1/1
  Low-Pass Filter (Discrete or Continuous)2/1 -> Iabc/1
  PS-Simulink Converter/1 -> Low-Pass Filter (Discrete or Continuous)2/1
  Low-Pass Filter (Discrete or Continuous)1/1 -> Vabc/1
  connections:
  PS-Simulink Converter1/LConn1 -- Phase Voltage Sensor (Three-Phase)/RConn1
  Phase Voltage Sensor (Three-Phase)/LConn1 -- Current Sensor (Three-Phase)/RConn2 -- Opabc/RConn1
  Current Sensor (Three-Phase)/LConn1 -- Inabc/RConn1
  PS-Simulink Converter/LConn1 -- Current Sensor (Three-Phase)/RConn1
  Phase Voltage Sensor (Three-Phase)/RConn2 -- Neutral Port (Three-Phase)/LConn1
  Electrical Reference1/LConn1 -- Neutral Port (Three-Phase)/RConn1

== system GridFormingConverter/Grid-Forming Converter/BusCalculations ==
  Vabc : Inport
  Iabc : Inport  Port=2
  Bus Creator : BusCreator  Inputs=6
  Bus Creator3 : BusCreator  Inputs=4
  Bus Creator4 : BusCreator  Inputs=4
  Complex2Phasor : Subsystem
  Complex2Phasor1 : Subsystem
  Demux : Demux  Outputs=3
  Demux1 : Demux  Outputs=3
  Measurement Unit (Phasor Computation) : Subsystem  mask(Measurement Unit){Ts=Ts}
      mask prompts: Ts "Sample time:"
  "Power (3ph, Instantaneous)1" : spsPower3phInstantaneousLib/Power (3ph, Instantaneous)
  SymmetricalComponentsCalc : Subsystem
  SymmetricalComponentsCalc1 : Subsystem
  BusCalcs : Outport
  wires:
  Vabc/1 -> Demux/1, Measurement Unit (Phasor Computation)/1(Vabc(t)), "Power (3ph, Instantaneous)1"/1
  Iabc/1 -> Demux1/1, Measurement Unit (Phasor Computation)/2(Iabc(t)), "Power (3ph, Instantaneous)1"/2
  "Power (3ph, Instantaneous)1"/2 -> Bus Creator/6  "Q"
  Measurement Unit (Phasor Computation)/2(" Iabc_Fund") -> SymmetricalComponentsCalc1/1(abc), Complex2Phasor1/1(complex)
  Demux1/1 -> Bus Creator4/1  "a"
  Bus Creator3/1 -> Bus Creator/1  "V"
  Demux/2 -> Bus Creator3/2  "b"
  Demux1/3 -> Bus Creator4/3  "c"
  Measurement Unit (Phasor Computation)/1(Vabc_Fund) -> Complex2Phasor/1(complex), SymmetricalComponentsCalc/1(abc)
  SymmetricalComponentsCalc1/1(ABC+-0) -> Bus Creator/4  "ISymm"
  Demux/1 -> Bus Creator3/1  "a"
  SymmetricalComponentsCalc/1(ABC+-0) -> Bus Creator/2  "VSymm"
  Bus Creator4/1 -> Bus Creator/3  "I"
  Demux1/2 -> Bus Creator4/2  "b"
  "Power (3ph, Instantaneous)1"/1 -> Bus Creator/5  "P"
  Demux/3 -> Bus Creator3/3  "c"
  Bus Creator/1 -> BusCalcs/1
  Complex2Phasor/1(Phasor) -> Bus Creator3/4  "Phasor"
  Complex2Phasor1/1(Phasor) -> Bus Creator4/4  "Phasor"

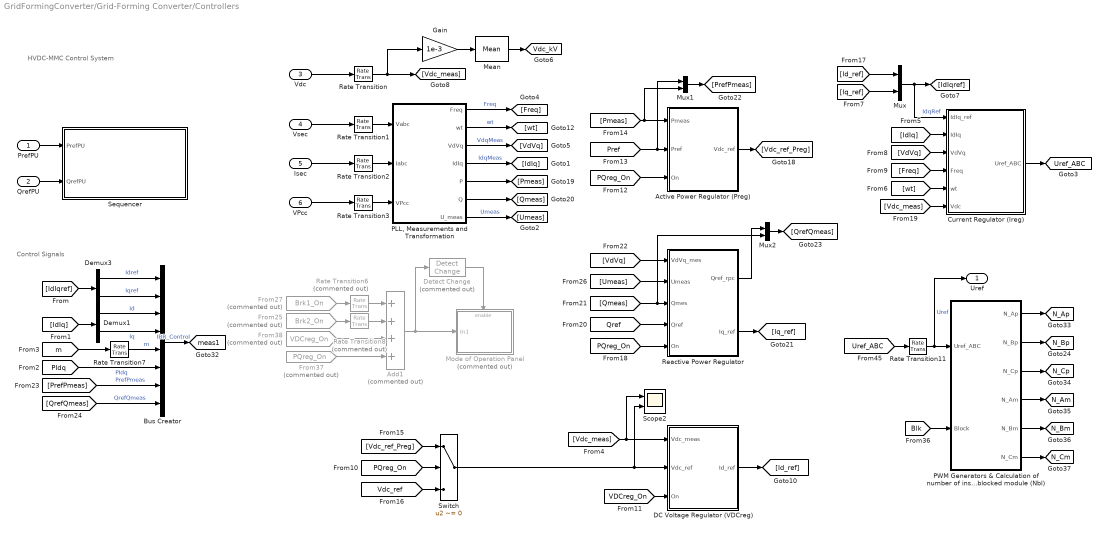
== system GridFormingConverter/Grid-Forming Converter/Controllers ==
  note: Control Signals
  note: HVDC-MMC Control System
  PrefPU : Inport
  QrefPU : Inport  Port=2
  Vdc : Inport  Port=3
  Vsec : Inport  Port=4
  Isec : Inport  Port=5
  VPcc : Inport  Port=6
  Active Power Regulator (Preg) : Subsystem
  Add1 : Sum  Commented=on  Inputs=++++
  Bus Creator : BusCreator  Inputs=8
  Current Regulator (Ireg) : Subsystem
  DC Voltage Regulator (VDCreg) : Subsystem
  Demux1 : Demux  Outputs=2
  Demux3 : Demux  Outputs=2
  Detect Change : simulink/Logic and Bit Operations/Detect Change  Commented=on  vinit=0  OutDataTypeStr=boolean
  From25 : From  Commented=on  GotoTag=Brk2_On  TagVisibility=global
  From27 : From  Commented=on  GotoTag=Brk1_On  TagVisibility=global
  From37 : From  Commented=on  GotoTag=PQreg_On  TagVisibility=global
  From38 : From  Commented=on  GotoTag=VDCreg_On  TagVisibility=global
  Gain : Gain  Gain=1e-3
  Mean : spsMeanLib/Mean  Freq=ConvCtrl.Freq/3  Vinit=0  Ts=ConvCtrl.Ts
  Mode of Operation Panel : Subsystem  Commented=on
  Mux : Mux  Inputs=2
  Mux1 : Mux  Inputs=2
  Mux2 : Mux  Inputs=2
  "PLL, Measurements and Transformation" : Subsystem
  PWM Generators & Calculation of number of inserted modules (Nin) and number of blocked module (Nbl) : Subsystem
  Rate Transition{,1..3,7} (5 alike) : RateTransition  OutPortSampleTime=ConvCtrl.Ts
  Rate Transition11 : RateTransition  OutPortSampleTime=PlantSim.Ts
  Rate Transition6 : RateTransition  Commented=on  OutPortSampleTime=ConvCtrl.Ts
  Rate Transition8 : RateTransition  Commented=on  OutPortSampleTime=ConvCtrl.Ts
  Reactive Power Regulator : Subsystem
  Scope2 : Scope  NumInputPorts=2
  Sequencer : Subsystem
      mask Display: disp('Sequencer')
  Switch : Switch  Criteria=u2 ~= 0  SaturateOnIntegerOverflow=off  InputSameDT=off
  Uref : Outport
  tag scope: N_Am=global, N_Ap=global, N_Bm=global, N_Bp=global, N_Cm=global, N_Cp=global, Uref_ABC=global, Vdc_kV=global, meas1=global
  wires:
  Reactive Power Regulator/1(Qref_rpc) -> Mux2/1
  [Umeas] -> Reactive Power Regulator/2(Umeas)
  "PLL, Measurements and Transformation"/7(U_meas) -> [Umeas]  "Umeas"
  Rate Transition3/1 -> "PLL, Measurements and Transformation"/3(VPcc)
  VPcc/1 -> Rate Transition3/1
  [Vdc_meas] -> DC Voltage Regulator (VDCreg)/1(Vdc_meas), Scope2/1
  Rate Transition11/1 -> PWM Generators & Calculation of number of inserted modules (Nin) and number of blocked module (Nbl)/1(Uref_ABC), Uref/1  "Uref"
  From27/1 -> Rate Transition6/1
  Rate Transition8/1 -> Add1/2
  From25/1 -> Rate Transition8/1
  From37/1 -> Add1/4
  From38/1 -> Add1/3
  Rate Transition6/1 -> Add1/1
  Add1/1 -> Detect Change/1, Mode of Operation Panel/1(In1)
  Detect Change/1 -> Mode of Operation Panel/Enable
  [Blk] -> PWM Generators & Calculation of number of inserted modules (Nin) and number of blocked module (Nbl)/2(Block)
  PWM Generators & Calculation of number of inserted modules (Nin) and number of blocked module (Nbl)/6(N_Cm) -> [N_Cm]
  PWM Generators & Calculation of number of inserted modules (Nin) and number of blocked module (Nbl)/5(N_Bm) -> [N_Bm]
  PWM Generators & Calculation of number of inserted modules (Nin) and number of blocked module (Nbl)/4(N_Am) -> [N_Am]
  PWM Generators & Calculation of number of inserted modules (Nin) and number of blocked module (Nbl)/3(N_Cp) -> [N_Cp]
  PWM Generators & Calculation of number of inserted modules (Nin) and number of blocked module (Nbl)/2(N_Bp) -> [N_Bp]
  PWM Generators & Calculation of number of inserted modules (Nin) and number of blocked module (Nbl)/1(N_Ap) -> [N_Ap]
  [Pmeas] -> Mux1/2, Active Power Regulator (Preg)/1(Pmeas)
  "PLL, Measurements and Transformation"/6(Q) -> [Qmeas]
  [PrefPmeas] -> Bus Creator/7  "PrefPmeas"
  [Pref] -> Mux1/1, Active Power Regulator (Preg)/2(Pref)
  Switch/1 -> DC Voltage Regulator (VDCreg)/2(Vdc_ref), Scope2/2
  [PQreg_On] -> Switch/2
  [Qmeas] -> Reactive Power Regulator/3(Qmes), Mux2/2
  [VdVq] -> Reactive Power Regulator/1(VdVq_mes)
  "PLL, Measurements and Transformation"/5(P) -> [Pmeas]
  Reactive Power Regulator/2(Iq_ref) -> [Iq_ref]
  Active Power Regulator (Preg)/1(Vdc_ref) -> [Vdc_ref_Preg]
  [PQreg_On] -> Active Power Regulator (Preg)/3(On)
  [VDCreg_On] -> DC Voltage Regulator (VDCreg)/3(On)
  [QrefQmeas] -> Bus Creator/8  "QrefQmeas"
  [Qref] -> Reactive Power Regulator/4(Qref)
  [Vdc_ref_Preg] -> Switch/1
  Mux1/1 -> [PrefPmeas]
  Mux2/1 -> [QrefQmeas]
  [PQreg_On] -> Reactive Power Regulator/5(On)
  [Vdc_ref] -> Switch/3
  Rate Transition1/1 -> "PLL, Measurements and Transformation"/1(Vabc)
  Rate Transition7/1 -> Bus Creator/5  "m"
  Rate Transition2/1 -> "PLL, Measurements and Transformation"/2(Iabc)
  Rate Transition/1 -> [Vdc_meas], Gain/1
  [Iq_ref] -> Mux/2
  [VdVq] -> Current Regulator (Ireg)/3(VdVq)
  "PLL, Measurements and Transformation"/1(Freq) -> [Freq]  "Freq"
  [PIdq] -> Bus Creator/6  "PIdq"
  Demux1/1 -> Bus Creator/3  "Id"
  [m] -> Rate Transition7/1
  Demux3/2 -> Bus Creator/2  "Iqref"
  Bus Creator/1 -> [meas1]  "IBR_Control"
  [IdIq] -> Demux1/1
  Demux3/1 -> Bus Creator/1  "Idref"
  [IdIqref] -> Demux3/1
  [IdIq] -> Current Regulator (Ireg)/2(IdIq)
  Demux1/2 -> Bus Creator/4  "Iq"
  Mux/1 -> [IdIqref], Current Regulator (Ireg)/1(IdIq_ref)  "IdqRef"
  "PLL, Measurements and Transformation"/3(VdVq) -> [VdVq]  "VdqMeas"
  [Id_ref] -> Mux/1
  [Freq] -> Current Regulator (Ireg)/4(Freq)
  "PLL, Measurements and Transformation"/4(IdIq) -> [IdIq]  "IdqMeas"
  "PLL, Measurements and Transformation"/2(wt) -> [wt]  "wt"
  Vdc/1 -> Rate Transition/1
  [wt] -> Current Regulator (Ireg)/5(wt)
  Current Regulator (Ireg)/1(Uref_ABC) -> [Uref_ABC]
  Gain/1 -> Mean/1
  DC Voltage Regulator (VDCreg)/1(Id_ref) -> [Id_ref]
  [Vdc_meas] -> Current Regulator (Ireg)/6(Vdc)
  Isec/1 -> Rate Transition2/1
  Vsec/1 -> Rate Transition1/1
  Mean/1 -> [Vdc_kV]
  [Uref_ABC] -> Rate Transition11/1
  PrefPU/1 -> Sequencer/1(PrefPU)
  QrefPU/1 -> Sequencer/2(QrefPU)

== system GridFormingConverter/Grid-Forming Converter/Grid-Forming Converter Control ==
  Pref : Inport
  Qref : Inport  Port=2
  Igabc : Inport  Port=3
  Vgabc : Inport  Port=4
  Current Limiting : Subsystem
  Grid Voltage Reactive Power Support : Subsystem
  Measurement : Subsystem
      mask Display: image('$imagefile'); % Use "Edit Image" on toolstrip to change.
  Power Control : Subsystem
  Rate Transition3 : RateTransition
  VoltageCurrentControl : Subsystem
      settings: PortSchema="{\"entries\":[{\"content\":{\"sides\":[{\"content\":{\"connectorIds\":[\"In1\",\"In2\"]},\"type\":\"ConnectorPlacement.EquallySpacedRectSide\",\"uuid\":\"0bf15a12-7bc0-47e4-89bd-435769673763\"},{\"content\":{\"connectorIds\":[\"Out1\"],\"side\":\"RIGHT\"},\"type\":\"ConnectorPlacement.EquallySpacedRectSide\",\"uuid\":\"44a15d74-8878-4ec6-abe4-be0b1b609519\"},{\"content\":{\"connectorIds\":[\"In3\"],\"side\":\"TOP\"},\"type\":\"ConnectorPlacement.EquallySpacedRectSide\",\"uuid\":\"7a96781e-5638-4b2a-8101-d5785aae9f0f\"}]},\"type\":\"ConnectorPlacement.EquallySpacedConnector\",\"uuid\":\"4b3373ad-cf20-4175-894e-3bd1604dd0ce\"}],\"packageUris\":[\"http://schema.mathworks.com/mf0/Connector/R2020b\"],\"version\":\"1.0\"}"
  mabc : Outport
  Pmeas : Outport  Port=2
  Qmeas : Outport  Port=3
  fmeas : Outport  Port=4
  wires:
  VoltageCurrentControl/1(mabc) -> mabc/1
  Vgabc/1 -> Measurement/1(Vgabcc)
  Igabc/1 -> Measurement/2(Igabc)
  Measurement/2(Pmeas) -> Pmeas/1
  Measurement/3(Qmeas) -> Qmeas/1
  Measurement/1(measure) -> Rate Transition3/1
  Power Control/3(angle) -> Measurement/3(Angle)
  Power Control/1(reactiveControl) -> Current Limiting/2(reactiveControl)
  Current Limiting/1(currentLimiting) -> VoltageCurrentControl/1(currentLimiting)
  Qref/1 -> Grid Voltage Reactive Power Support/3(QrefInput)
  Pref/1 -> Grid Voltage Reactive Power Support/2(PrefInput)
  Grid Voltage Reactive Power Support/1(Pref) -> Power Control/2(Pref)
  Grid Voltage Reactive Power Support/2(Qref) -> Power Control/3(Qref)
  Measurement/4(fmeas) -> fmeas/1
  Rate Transition3/1 -> Current Limiting/1(measure), VoltageCurrentControl/3(measure), Power Control/1(measure), Grid Voltage Reactive Power Support/1(measure)
  Power Control/2(activeControl) -> VoltageCurrentControl/2(activeControl)

== system GridFormingConverter/Grid-Forming Converter/Grid-Forming Converter Power Circuit ==
  mabc : Inport
  Filter & Sensor : Subsystem
      mask Display: image('$imagefile'); % Use "Edit Image" on toolstrip to change.
  Grid Forming Converter : ee_lib/Semiconductors & Converters/Converters/Average-Value Voltage Source Converter (Three-Phase)  port_option=ee.enum.threePhasePort.composite  frequency_option=ee.enum.converters.frequency.variable  input_option=ee.enum.converters.inputOption.ModWave  FRated=50 Hz  losses_parameterization=ee.enum.converters.losses.fixed  Pfixed=10 W  ks=0.01  kc1=1.7 V  kc2=0.01 Ohm  Ploss_vect=[100, 800, 1870, 3250, 4900] W  Irms_vect=[10, 100, 200, 300, 400] A  Vdc_nom=300 V  thermal_mass=30000 J/K  temperature_specify=off  temperature_priority=High  temperature=298.15 K  temperature_nominal_specify=off  temperature_nominal_value=1  temperature_nominal_unit=K
      settings: InternalSimscapePortConfiguration="{\"Bottom\":[],\"Left\":[{\"id\":\"ModWave\",\"label\":\"ModWave\",\"type\":\"input\"},{\"id\":\"N\",\"label\":\"~\",\"type\":\"foundation.electrical.three_phase\"}],\"Right\":[{\"id\":\"p\",\"label\":\"+\",\"type\":\"foundation.electrical.electrical\"},{\"id\":\"n\",\"label\":\"-\",\"type\":\"foundation.electrical.electrical\"}],\"Top\":[]}"
  Simulink-PS Converter : nesl_utility/Simulink-PS Converter  PhysicalDomain=network_engine_domain  SubClassName=ps_input  LeftPortType=input  RightPortType=output  PseudoPeriodic=off  Frequencies=[]  NoiseDistribution=none  NoiseParameters=[]  Unit=1  AffineConversion=off  FilteringAndDerivatives=provide  SimscapeFilterOrder=1  InputFilterTimeConstant=0.001  UdotUserProvided=0
  P : PMIOPort  Side=Left
  N : PMIOPort  Port=2  Side=Left
  ABC : PMIOPort  Port=3  Side=Right
  Iabc : Outport
  Vabc : Outport  Port=2
  wires:
  mabc/1 -> Simulink-PS Converter/1
  Filter & Sensor/1(Iabc) -> Iabc/1
  Filter & Sensor/2(Vabc) -> Vabc/1
  connections:
  Grid Forming Converter/LConn2 -- Filter & Sensor/LConn1
  Simulink-PS Converter/RConn1 -- Grid Forming Converter/LConn1
  P/RConn1 -- Grid Forming Converter/RConn1
  ABC/RConn1 -- Filter & Sensor/RConn1
  Grid Forming Converter/RConn2 -- N/RConn1

== system GridFormingConverter/Transformer 415 V//11 kV/Filter & Sensor ==
  Current Sensor (Three-Phase) : ee_lib/Sensors & Transducers/Current Sensor (Three-Phase)
  Electrical Reference1 : fl_lib/Electrical/Electrical Elements/Electrical Reference
  Low-Pass Filter (Discrete or Continuous)1 : eeGeneralControl/Low-Pass Filter (Discrete or Continuous)  K=1  T=1/(200*gridInverter.frequency)  B=inf  A=-inf  init_option=Specify as parameter  x0=0  Ts=gridInverter.controller.VoltageControlSampleTime
  Low-Pass Filter (Discrete or Continuous)2 : eeGeneralControl/Low-Pass Filter (Discrete or Continuous)  K=1  T=1/(200*gridInverter.frequency)  B=inf  A=-inf  init_option=Specify as parameter  x0=0  Ts=gridInverter.controller.VoltageControlSampleTime
  Neutral Port (Three-Phase) : ee_lib/Connectors & References/Neutral Port (Three-Phase)  G_parasitic=1e-12 1/Ohm
      settings: InternalSimscapePortConfiguration="{\"Bottom\":[],\"Left\":[{\"id\":\"N\",\"label\":\"~\",\"type\":\"foundation.electrical.three_phase\"}],\"Right\":[{\"id\":\"n\",\"label\":\"n\",\"type\":\"foundation.electrical.electrical\"}],\"Top\":[]}"
  PS-Simulink Converter : nesl_utility/PS-Simulink Converter  PhysicalDomain=network_engine_domain  SubClassName=ps_output  LeftPortType=input  RightPortType=output  PseudoPeriodic=off  Frequencies=[]  VectorFormat=inherit  Unit=inherit  AffineConversion=off
  PS-Simulink Converter1 : nesl_utility/PS-Simulink Converter  PhysicalDomain=network_engine_domain  SubClassName=ps_output  LeftPortType=input  RightPortType=output  PseudoPeriodic=off  Frequencies=[]  VectorFormat=inherit  Unit=inherit  AffineConversion=off
  Phase Voltage Sensor (Three-Phase) : ee_lib/Sensors & Transducers/Phase Voltage Sensor (Three-Phase)
  Inabc : PMIOPort  Side=Left
  Opabc : PMIOPort  Port=2  Side=Right
  Iabc : Outport
  Vabc : Outport  Port=2
  wires:
  PS-Simulink Converter1/1 -> Low-Pass Filter (Discrete or Continuous)1/1
  Low-Pass Filter (Discrete or Continuous)2/1 -> Iabc/1
  PS-Simulink Converter/1 -> Low-Pass Filter (Discrete or Continuous)2/1
  Low-Pass Filter (Discrete or Continuous)1/1 -> Vabc/1
  connections:
  PS-Simulink Converter1/LConn1 -- Phase Voltage Sensor (Three-Phase)/RConn1
  Current Sensor (Three-Phase)/LConn1 -- Inabc/RConn1
  PS-Simulink Converter/LConn1 -- Current Sensor (Three-Phase)/RConn1
  Phase Voltage Sensor (Three-Phase)/LConn1 -- Current Sensor (Three-Phase)/RConn2 -- Opabc/RConn1
  Phase Voltage Sensor (Three-Phase)/RConn2 -- Neutral Port (Three-Phase)/LConn1
  Electrical Reference1/LConn1 -- Neutral Port (Three-Phase)/RConn1
